simulink model "run_external_mode"  (R2025b)
settings: Solver=FixedStepAuto  StartTime=0.0  StopTime=10.0  FixedStep=0.02  RelTol=1e-3
values from neighbouring files (symbols this model uses):
  inputs = sscanf(dataStr, '    [run_controller.m]
settings Model: Creator=schwmaxi  LastModifiedBy=schwmaxi
settings OptimizationCC: UseDivisionForNetSlopeComputation=on  DefaultUnderspecifiedDataType=single

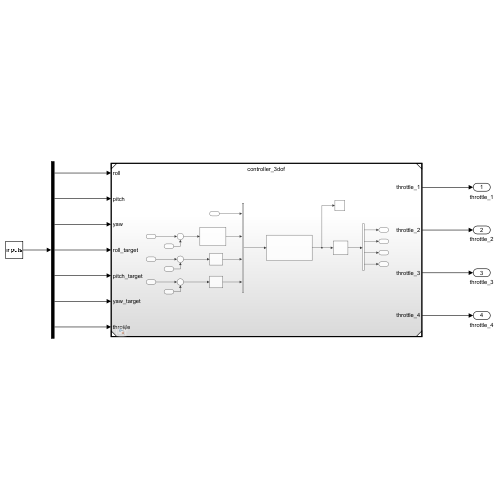
[thumbnail: Simulink's stored preview of the top-level diagram]
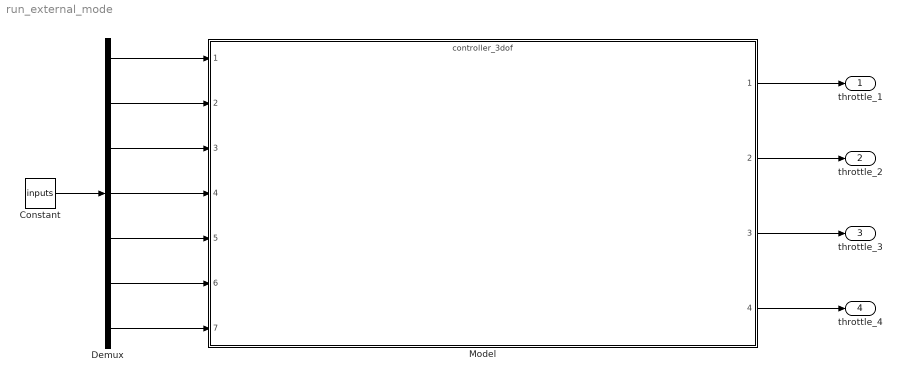
== system run_external_mode ==
  Constant : Constant  Value=inputs
  Demux : Demux  Outputs=7
  Model : ModelReference  ModelNameDialog=controller_3dof.slx  SimulationMode=Normal  ModelReferenceVersion=1.118
  throttle_1 : Outport
  throttle_2 : Outport  Port=2
  throttle_3 : Outport  Port=3
  throttle_4 : Outport  Port=4
  wires:
  Demux/1 -> Model/1
  Demux/2 -> Model/2
  Demux/3 -> Model/3
  Demux/4 -> Model/4
  Demux/5 -> Model/5
  Demux/6 -> Model/6
  Demux/7 -> Model/7
  Constant/1 -> Demux/1
  Model/1 -> throttle_1/1
  Model/2 -> throttle_2/1
  Model/4 -> throttle_4/1
  Model/3 -> throttle_3/1
